simulink model "Project7SimulinkPID"  (R2020a)
settings: Solver=VariableStepAuto  StartTime=0.0  StopTime=10.0  RelTol=1e-3
values from neighbouring files (symbols this model uses):
  kd = 10    [Project7.m]
  ki = 5    [Project7.m]
  kp = 350    [Project7.m]
settings Model: Creator=cresp  LastModifiedBy=cresp

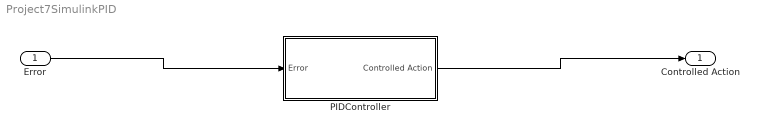
== system Project7SimulinkPID ==
  Error : Inport
  PIDController : Subsystem
  Controlled Action : Outport
  wires:
  Error/1 -> PIDController/1(Error)
  PIDController/1(Controlled Action) -> Controlled Action/1

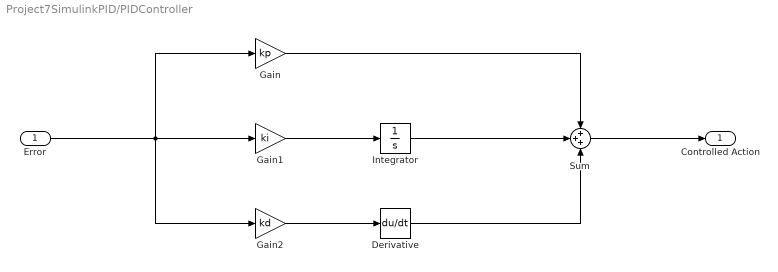
== system Project7SimulinkPID/PIDController ==
  Error : Inport
  Derivative : Derivative
  Gain : Gain  Gain=kp
  Gain1 : Gain  Gain=ki
  Gain2 : Gain  Gain=kd
  Integrator : Integrator
  Sum : Sum  Inputs=+++
  Controlled Action : Outport
  wires:
  Sum/1 -> Controlled Action/1
  Error/1 -> Gain/1, Gain1/1, Gain2/1
  Gain1/1 -> Integrator/1
  Gain/1 -> Sum/1
  Derivative/1 -> Sum/3
  Integrator/1 -> Sum/2
  Gain2/1 -> Derivative/1
